simulink model "three_phase_mulitslx"  (R2024a)
settings: Solver=VariableStepAuto  StartTime=0.0  StopTime=5  RelTol=1e-3
undefined symbols (not defined in the file): D1, Delta
libraries: spsDiodeLib x12, spsCurrentMeasurementLib x8, spsSeriesRLCBranchLib x5, spsACVoltageSourceLib x3, spsThreePhaseTransformerThreeWindingsLib x1, spsVoltageMeasurementLib x1, sps_lib x1
settings Model: Creator=farza  LastModifiedBy=farza
settings DataIOCC: ReturnWorkspaceOutputs=off

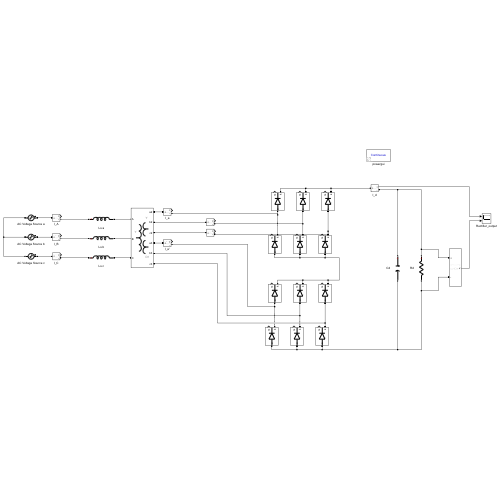
[thumbnail: Simulink's stored preview of the top-level diagram]
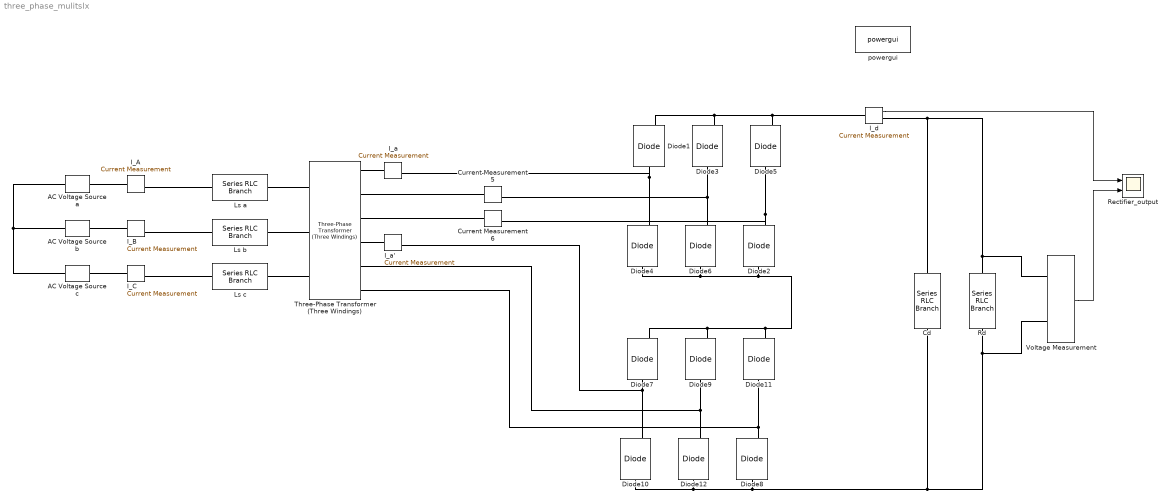
== system three_phase_mulitslx ==
  AC Voltage Source a : spsACVoltageSourceLib/AC Voltage Source  Amplitude=4160  Phase=0  Frequency=60  SampleTime=0  Measurements=None  BusType=swing  Pref=10e3  Qref=0  Qmin=-inf  Qmax=+inf
  AC Voltage Source b : spsACVoltageSourceLib/AC Voltage Source  Amplitude=4160  Phase=120  Frequency=60  SampleTime=0  Measurements=None  BusType=swing  Pref=10e3  Qref=0  Qmin=-inf  Qmax=+inf
  AC Voltage Source c : spsACVoltageSourceLib/AC Voltage Source  Amplitude=4160  Phase=240  Frequency=60  SampleTime=0  Measurements=None  BusType=swing  Pref=10e3  Qref=0  Qmin=-inf  Qmax=+inf
  Cd : spsSeriesRLCBranchLib/Series RLC Branch  LConnTagsString=__new0  RConnTagsString=__new0  BranchType=C  Resistance=1  Inductance=0  SetiL0=off  InitialCurrent=0  Capacitance=2e-2  Setx0=off  InitialVoltage=0  Measurements=None
  Current Measurement5 : spsCurrentMeasurementLib/Current Measurement  PhasorSimulation=off  OutputType=Complex  PSBequivalent=0
  Current Measurement6 : spsCurrentMeasurementLib/Current Measurement  PhasorSimulation=off  OutputType=Complex  PSBequivalent=0
  Diode{1..3,5,7..9,11} (8 alike) : spsDiodeLib/Diode  Ron=0  Lon=0  Vf=0.8  IC=0  UseSnubber=0  Rs=0  Cs=0  Measurements=on
  Diode{4,6,10,12} (4 alike) : spsDiodeLib/Diode  Ron=0  Lon=0  Vf=0  IC=0  UseSnubber=0  Rs=0  Cs=0  Measurements=on
  I_A : spsCurrentMeasurementLib/Current Measurement  PhasorSimulation=off  OutputType=Complex  PSBequivalent=0
  I_B : spsCurrentMeasurementLib/Current Measurement  PhasorSimulation=off  OutputType=Complex  PSBequivalent=0
  I_C : spsCurrentMeasurementLib/Current Measurement  PhasorSimulation=off  OutputType=Complex  PSBequivalent=0
  I_a : spsCurrentMeasurementLib/Current Measurement  PhasorSimulation=off  OutputType=Complex  PSBequivalent=0
  I_a' : spsCurrentMeasurementLib/Current Measurement  PhasorSimulation=off  OutputType=Complex  PSBequivalent=0
  I_d : spsCurrentMeasurementLib/Current Measurement  PhasorSimulation=off  OutputType=Complex  PSBequivalent=0
  Ls a : spsSeriesRLCBranchLib/Series RLC Branch  LConnTagsString=__new0  RConnTagsString=__new0  BranchType=L  Resistance=1  Inductance=2.295e-3  SetiL0=off  InitialCurrent=0  Capacitance=1e-6  Setx0=off  InitialVoltage=0  Measurements=None
  Ls b : spsSeriesRLCBranchLib/Series RLC Branch  LConnTagsString=__new0  RConnTagsString=__new0  BranchType=L  Resistance=1  Inductance=2.295e-3  SetiL0=off  InitialCurrent=0  Capacitance=1e-6  Setx0=off  InitialVoltage=0  Measurements=None
  Ls c : spsSeriesRLCBranchLib/Series RLC Branch  LConnTagsString=__new0  RConnTagsString=__new0  BranchType=L  Resistance=1  Inductance=2.295e-3  SetiL0=off  InitialCurrent=0  Capacitance=1e-6  Setx0=off  InitialVoltage=0  Measurements=None
  Rd : spsSeriesRLCBranchLib/Series RLC Branch  LConnTagsString=__new0  RConnTagsString=__new0  BranchType=R  Resistance=0.25  Inductance=0  SetiL0=off  InitialCurrent=0  Capacitance=1e-6  Setx0=off  InitialVoltage=0  Measurements=None
  Rectifier_output : Scope  NumInputPorts=2
  Three-Phase Transformer (Three Windings) : spsThreePhaseTransformerThreeWindingsLib/Three-Phase Transformer (Three Windings)  Winding1Connection=Y  Winding2Connection=Y  Winding3Connection=Delta (D1)  CoreType=Three single-phase transformers  SetSaturation=off  Hysteresis=off  DataFile='hysteresis'  SetInitialFlux=off  Measurements=None  UNITS=pu  NominalPower=[ 1e9 , 60 ]  Winding1=[4160, 0, 0.03]  Winding2=[2102, 0, 0.03]  Winding3=[2102, 0, 0.03]  Rm=10  Lm=10  L0=0.5  Saturation=[0 0;0.0024 1.2;1 1.52]  InitialFluxes=[0.8 -0.8 0.7]  BreakLoop=off  DiscreteSolver=Trapezoidal iterative  DataType=off  TransfoNumber=1
      settings: LibrarySourceBlock=|
      | sps_lib/Power Grid Elements/Three-Phase
      | Transformer
      | (Three Windings)
  Voltage Measurement : spsVoltageMeasurementLib/Voltage Measurement  PhasorSimulation=off  OutputType=Complex  PSBequivalent=0
  powergui : sps_lib/powergui  Priority=1  SimulationMode=Continuous  SampleTime=50e-6  frequency=60  Iterations=50  frequencyindice=60  Pbase=100e6  ErrMax=1e-4  UnitsV=kV  UnitsW=MW  buscounter=0  FunctionMessages=off  echomessages=off  EnableUseOfTLC=off  CurrentSourceSwitches=off  DisableSnubberDevices=off  DisableRonSwitches=off  DisableVfSwitches=off  DisplayEquations=off  AutomaticDiscreteSolvers=off  SolverType=Tustin/Backward Euler (TBE)  Interpol=off  ExternalGateDelay=off  methode=off  Ts=100  x0status=blocks  SPID=on  SwTol=0  HookPort=off  NonlinearTolerance=1e-4  nMaxIteration=100  ContinueOnMaxIteration=off  RestoreLinks=warning  ResistiveCurrentMeasurement=off  Frange=[0:2:500]  Ylog=off  Xlog=on  ShowGrid=off  save=off  variable=ZData  structure=A_Currents  ZoomFFT=off  StartTime=0  cycles=1  DisplayStyle=1  fundamental=60  FreqAxis=off  MaxFrequency=2000  frequencyindicesteady=1  RmsSteady=1  display=off
  wires:
  Voltage Measurement/1 -> Rectifier_output/2
  I_d/1 -> Rectifier_output/1
  connections:
  Diode1/LConn1 -- Diode4/RConn1 -- I_a/RConn1
  Rd/LConn1 -- I_d/RConn1 -- Cd/LConn1 -- Voltage Measurement/LConn1
  Diode11/LConn1 -- Diode8/RConn1 -- Three-Phase Transformer (Three Windings)/RConn6
  Diode10/LConn1 -- Cd/RConn1 -- Rd/RConn1 -- Voltage Measurement/LConn2 -- Diode8/LConn1 -- Diode12/LConn1
  Diode4/LConn1 -- Diode6/LConn1 -- Diode2/LConn1 -- Diode9/RConn1 -- Diode7/RConn1 -- Diode11/RConn1
  Diode5/LConn1 -- Diode2/RConn1 -- Current Measurement6/RConn1
  Diode1/RConn1 -- Diode5/RConn1 -- I_d/LConn1 -- Diode3/RConn1
  AC Voltage Source b/LConn1 -- AC Voltage Source a/LConn1 -- AC Voltage Source c/LConn1
  Diode6/RConn1 -- Diode3/LConn1 -- Current Measurement5/RConn1
  Diode9/LConn1 -- Diode12/RConn1 -- Three-Phase Transformer (Three Windings)/RConn5
  Diode10/RConn1 -- Diode7/LConn1 -- I_a'/RConn1
  AC Voltage Source a/RConn1 -- I_A/LConn1
  Current Measurement6/LConn1 -- Three-Phase Transformer (Three Windings)/RConn3
  I_a'/LConn1 -- Three-Phase Transformer (Three Windings)/RConn4
  I_C/RConn1 -- Ls c/LConn1
  AC Voltage Source c/RConn1 -- I_C/LConn1
  Current Measurement5/LConn1 -- Three-Phase Transformer (Three Windings)/RConn2
  I_a/LConn1 -- Three-Phase Transformer (Three Windings)/RConn1
  Ls c/RConn1 -- Three-Phase Transformer (Three Windings)/LConn3
  Ls b/RConn1 -- Three-Phase Transformer (Three Windings)/LConn2
  Ls a/RConn1 -- Three-Phase Transformer (Three Windings)/LConn1
  I_B/RConn1 -- Ls b/LConn1
  AC Voltage Source b/RConn1 -- I_B/LConn1
  I_A/RConn1 -- Ls a/LConn1
